simulink model "InertiaWheelSystemSATURATION"
settings: Solver=ode45  StartTime=0.0  StopTime=10.0  RelTol=1e-3
values from neighbouring files (symbols this model uses):
  A = [0 1 0; a/Jw 0 0 ; -(a/Jp) 0 0]    [modelFLAWED.m]
  B = [B_tau B_d]    [modelFLAWED.m]
  C = [1 0 0]    [modelFLAWED.m]
  D = 0    [modelFLAWED.m]
undefined symbols (not defined in the file or in its folder): ki, Kt, N, Tdt, Tit, x10, x20, x30
libraries: simulink x6, cstblocks x2, dspmtrx3 x1
settings Model: Creator=elt11jke  LastModifiedBy=frt090_B
settings DataIOCC: LimitDataPoints=on  SaveFormat=Array  SignalLoggingSaveFormat=ModelDataLogs  ReturnWorkspaceOutputs=off
settings OptimizationCC: ExpressionDepthLimit=2147483647  LifeSpan=inf  SimCompilerOptimization=Off
settings DebuggingCC: UnderspecifiedInitializationDetection=Classic  MergeDetectMultiDrivingBlocksExec=none  SolverPrmCheckMsg=warning  MultiTaskDSMMsg=warning  MultiTaskCondExecSysMsg=none  FcnCallInpInsideContextMsg=Enable All  FrameProcessingCompatibilityMsg=warning  StateNameClashWarn=warning  StrictBusMsg=None  SFUnexpectedBacktrackingDiag=warning  SFNoUnconditionalDefaultTransitionDiag=warning
settings HardwareCC: ProdBitPerPointer=32  ProdLargestAtomicFloat=None  ProdIntDivRoundTo=Undefined  ProdEndianess=Unspecified  ProdWordSize=32  ProdHWDeviceType=32-bit Generic
settings ModelReferenceCC: PropagateSignalLabelsOutOfModel=off
settings SFSimCC: SimUseLocalCustomCode=off
settings RTWCC: RTWUseLocalCustomCode=off  IncludeERTFirstTime=on  RTWCompilerOptimization=Off
settings GRTTargetCC: GeneratePreprocessorConditionals=Disable all

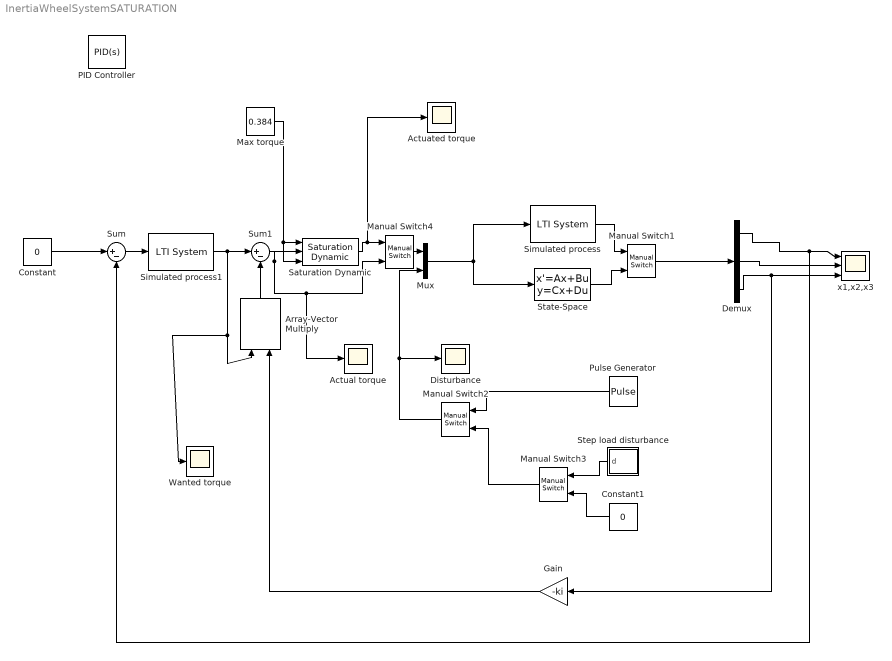
== system InertiaWheelSystemSATURATION ==
  Actual torque : Scope
      settings: ShowLegends=on  TimeRange=10  YMin=-200  YMax=-20
  Actuated torque : Scope
      settings: ShowLegends=on  TimeRange=10  YMin=0.384  YMax=0.384  SaveName=ScopeData4
  Array-Vector Multiply : dspmtrx3/Array-Vector Multiply  mode=Mute  saveAsFlag=0  Dimension=1  V_Source=Input port  V_VectFromMask=[0.5 0.25]  firstCoeffSignedness=Auto  firstCoeffDataTypeStr=Inherit: Same word length as input  firstCoeffLastDataTypeStr=Inherit: Same word length as input  firstCoeffMin=[]  firstCoeffMax=[]  outputSignedness=Auto  outputDataTypeStr=Inherit: Same as product output  outputLastDataTypeStr=Inherit: Same as product output  outputMin=[]  outputMax=[]  accumSignedness=Auto  prodOutputSignedness=Auto  roundingMode=Floor  overflowMode=off
  Constant : Constant  Value=0
  Constant1 : Constant  Value=0
  Demux : Demux  Outputs=3
  Disturbance : Scope
      settings: ShowLegends=on  TimeRange=10  YMin=-0.01  YMax=0.02  SaveName=ScopeData2
  Gain : Gain  Gain=-ki
  Manual Switch1 : simulink/Signal Routing/Manual Switch  sw=0  action=0  varsize=off
  Manual Switch2 : simulink/Signal Routing/Manual Switch  sw=0  action=0  varsize=off
  Manual Switch3 : simulink/Signal Routing/Manual Switch  sw=0  action=0  varsize=off
  Manual Switch4 : simulink/Signal Routing/Manual Switch  sw=1  action=0  varsize=off
  Max torque : Constant  Value=0.384
  Mux : Mux  Inputs=2
  PID Controller : simulink/Continuous/PID Controller  Controller=PID  TimeDomain=Continuous-time  SampleTime=1  IntegratorMethod=Forward Euler  FilterMethod=Forward Euler  Form=Parallel  P=Kt  I=Tit  D=Tdt  N=N  InitialConditionSource=internal  InitialConditionForIntegrator=0  InitialConditionForFilter=0  ExternalReset=none  LimitOutput=off  UpperSaturationLimit=inf  LowerSaturationLimit=-inf  LinearizeAsGain=off  AntiWindupMode=none  Kb=1  TrackingMode=off  Kt=1  PParamMin=[]  PParamMax=[]  IParamMin=[]  IParamMax=[]  DParamMin=[]  DParamMax=[]  NParamMin=[]  NParamMax=[]  KbParamMin=[]  KbParamMax=[]  KtParamMin=[]  KtParamMax=[]  POutMin=[]  POutMax=[]  IOutMin=[]  IOutMax=[]  DOutMin=[]  DOutMax=[]  NOutMin=[]  NOutMax=[]  KbOutMin=[]  KbOutMax=[]  KtOutMin=[]  KtOutMax=[]  IntegratorOutMin=[]  IntegratorOutMax=[]  FilterOutMin=[]  FilterOutMax=[]  SumOutMin=[]  SumOutMax=[]  SumI1OutMin=[]  SumI1OutMax=[]  SumI2OutMin=[]  SumI2OutMax=[]  SumI3OutMin=[]  SumI3OutMax=[]  SumDOutMin=[]  SumDOutMax=[]  SaturationOutMin=[]  SaturationOutMax=[]  IntegratorContinuousStateAttributes=''  IntegratorStateMustResolveToSignalObject=off  IntegratorRTWStateStorageClass=Auto  FilterContinuousStateAttributes=''  FilterStateMustResolveToSignalObject=off  FilterRTWStateStorageClass=Auto
  Pulse Generator : DiscretePulseGenerator  PulseType=Time based  Amplitude=0.01  Period=3  PulseWidth=5
  Saturation Dynamic : simulink/Discontinuities/Saturation Dynamic  OutMin=[-1]  OutMax=[1]  OutDataTypeStr=Inherit: Same as second input  OutDataType=fixdt(1, 16)  OutScaling=2^-10  DoSatur=off
  Simulated process : cstblocks/LTI System  sys=PinSF  IC=[]
  Simulated process1 : cstblocks/LTI System  sys=Cin  IC=[]
  State-Space : StateSpace  A=A  B=B  C=C  D=D  X0=[x10 x20 x30]
  Step load disturbance : Subsystem
  Sum : Sum  Inputs=|+-
  Sum1 : Sum  Inputs=|+-
  Wanted torque : Scope
      settings: ShowLegends=on  TimeRange=10  YMin=-1.355e+07  YMax=-1.3275e+07  SaveName=ScopeData3
  x1,x2,x3 : Scope  NumInputPorts=3
      settings: ShowLegends=on  TimeRange=10  YMin=1000~0~-0.0003  YMax=10000~90000~-2.5e-05
  wires:
  Constant/1 -> Sum/1
  Demux/1 -> x1,x2,x3/1, Sum/2
  Demux/2 -> x1,x2,x3/2
  Pulse Generator/1 -> Manual Switch2/1
  Manual Switch2/1 -> Mux/2, Disturbance/1
  Sum/1 -> Simulated process1/1
  Mux/1 -> State-Space/1, Simulated process/1
  Manual Switch1/1 -> Demux/1
  Step load disturbance/1(d) -> Manual Switch3/1
  Constant1/1 -> Manual Switch3/2
  Manual Switch3/1 -> Manual Switch2/2
  Simulated process/1 -> Manual Switch1/1
  State-Space/1 -> Manual Switch1/2
  Demux/3 -> x1,x2,x3/3, Gain/1
  Array-Vector Multiply/1 -> Sum1/2
  Gain/1 -> Array-Vector Multiply/2
  Max torque/1 -> Saturation Dynamic/1, Saturation Dynamic/3
  Simulated process1/1 -> Sum1/1, Array-Vector Multiply/1, Wanted torque/1
  Manual Switch4/1 -> Mux/1
  Saturation Dynamic/1 -> Manual Switch4/1, Actuated torque/1
  Sum1/1 -> Saturation Dynamic/2, Manual Switch4/2, Actual torque/1

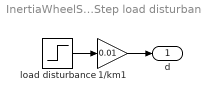
== system InertiaWheelSystemSATURATION/Step load disturbance ==
  1/km1 : Gain  Gain=0.01  SaturateOnIntegerOverflow=on  OutDataTypeStr=Inherit: Same as input  ParamDataTypeStr=Inherit: Same as input
  load disturbance : Step  Time=5  After=-0.15  SampleTime=0
  d : Outport
  wires:
  load disturbance/1 -> 1/km1/1
  1/km1/1 -> d/1
